simulink model "dynsim_2link_planar"  (R2020a)
settings: Solver=ode3  StartTime=0.0  StopTime=10.0  FixedStep=0.05  RelTol=1e-3
values from neighbouring files (symbols this model uses):
  L1 = 0.337    [dynsim_test_urdf_init.m]    (also in init_2link_planar.m)
  L2 = 0.210    (= 0.21)    [dynsim_test_urdf_init.m]    (also in init_2link_planar.m)
  L3 = 0.268    [dynsim_test_urdf_init.m]    (also in init_2link_planar.m)
  L4 = 0    [dynsim_test_urdf_init.m]    (also in init_2link_planar.m)
  L5 = 0.174    [dynsim_test_urdf_init.m]    (also in init_2link_planar.m)
  L6 = 0    [dynsim_test_urdf_init.m]    (also in init_2link_planar.m)
libraries: robotlib x18, robotmaniplib x1
settings Model: Creator=bascetta  LastModifiedBy=giulio
settings OptimizationCC: EnhancedBackFolding=on  PassReuseOutputArgsAs=Individual arguments  ZeroExternalMemoryAtStartup=off  ZeroInternalMemoryAtStartup=off  MaxStackSize=64  OptimizeBlockOrder=speed  DifferentSizesBufferReuse=on  OptimizationCustomize=off  EfficientTunableParamExpr=on
settings DebuggingCC: ParameterTunabilityLossMsg=error
settings HardwareCC: ProdBitPerPointer=32  ProdBitPerSizeT=32  ProdBitPerPtrDiffT=32  ProdLargestAtomicFloat=None  ProdIntDivRoundTo=Undefined  ProdEndianess=Unspecified  ProdWordSize=32  ProdHWDeviceType=Generic->Unspecified (assume 32-bit Generic)
settings RTWCC: SystemTargetFile=ert.tlc  HardwareBoard=Robot Operating System (ROS)  TemplateMakefile=ert_default_tmf  GenerateReport=on  Toolchain=Catkin  IncludeHyperlinkInReport=on  LaunchReport=on  TargetLang=C++  GenerateTraceInfo=on  GenerateTraceReport=on  GenerateTraceReportSl=on  GenerateTraceReportSf=on  GenerateTraceReportEml=on
settings CodeAppCC: ForceParamTrailComments=on  IgnoreCustomStorageClasses=off  OperatorAnnotations=on  SimulinkDataObjDesc=on  SFDataObjDesc=on  InsertBlockDesc=on
settings ERTTargetCC: SupportContinuousTime=on  SupportVariableSizeSignals=on

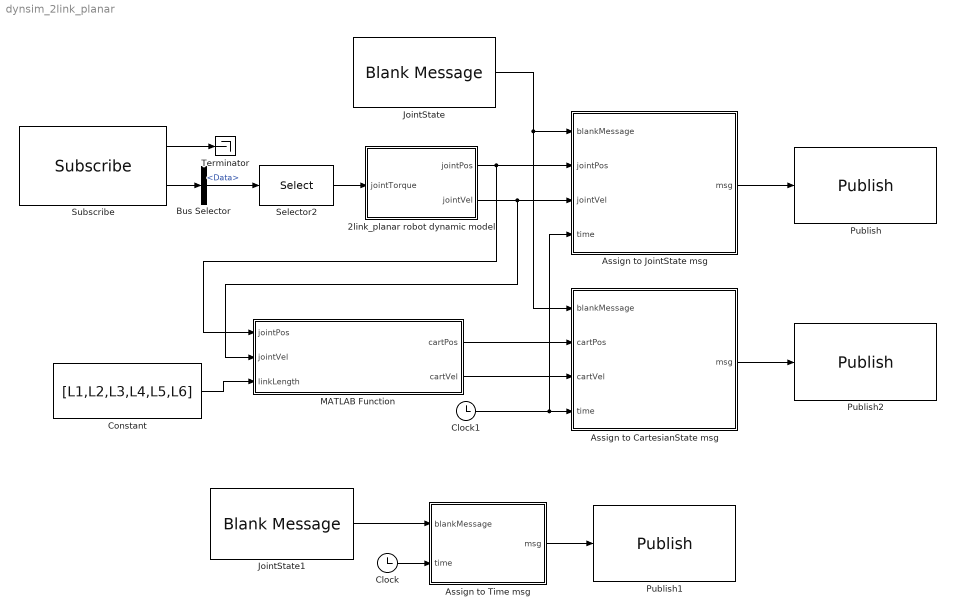
== system dynsim_2link_planar ==
  2link_planar robot dynamic model : Subsystem
  Assign to CartesianState msg : MATLAB Function  TreatAsAtomicUnit=on
  Assign to JointState msg : MATLAB Function  TreatAsAtomicUnit=on
  Assign to Time msg : MATLAB Function  TreatAsAtomicUnit=on
  Bus Selector : BusSelector  OutputSignals=Data
  Clock : Clock
  Clock1 : Clock
  Constant : Constant  Value=[L1,L2,L3,L4,L5,L6]
  JointState : robotlib/Blank Message  messageClass=Message  entityType=sensor_msgs/JointState  messageType=sensor_msgs/JointState  SampleTime=inf
  JointState1 : robotlib/Blank Message  messageClass=Message  entityType=rosgraph_msgs/Clock  messageType=rosgraph_msgs/Clock  SampleTime=inf
  MATLAB Function : MATLAB Function  TreatAsAtomicUnit=on
  Publish : robotlib/Publish  topicSource=Specify your own  topic=/edo/joint_states  messageType=sensor_msgs/JointState  messageQueueLength=1
  Publish1 : robotlib/Publish  topicSource=Specify your own  topic=/clock  messageType=rosgraph_msgs/Clock  messageQueueLength=1
  Publish2 : robotlib/Publish  topicSource=Specify your own  topic=/cartesian_states  messageType=sensor_msgs/JointState  messageQueueLength=1
  Selector2 : Selector  IndexOptions=Starting index (dialog)  Indices=[2]  OutputSizes=6
  Subscribe : robotlib/Subscribe  topicSource=Specify your own  topic=/joint_torque  messageType=std_msgs/Float64MultiArray  sampleTime=-1  messageQueueLength=1
  Terminator : Terminator
  wires:
  JointState1/1 -> Assign to Time msg/1(blankMessage)
  Assign to Time msg/1(msg) -> Publish1/1
  Subscribe/2 -> Bus Selector/1
  Subscribe/1 -> Terminator/1
  Selector2/1 -> 2link_planar robot dynamic model/1(jointTorque)
  Assign to JointState msg/1(msg) -> Publish/1
  2link_planar robot dynamic model/2(jointVel) -> MATLAB Function/2(jointVel), Assign to JointState msg/3(jointVel)
  Bus Selector/1 -> Selector2/1  "<Data>"
  2link_planar robot dynamic model/1(jointPos) -> MATLAB Function/1(jointPos), Assign to JointState msg/2(jointPos)
  Clock/1 -> Assign to Time msg/2(time)
  Clock1/1 -> Assign to CartesianState msg/4(time), Assign to JointState msg/4(time)
  MATLAB Function/2(cartVel) -> Assign to CartesianState msg/3(cartVel)
  Assign to CartesianState msg/1(msg) -> Publish2/1
  Constant/1 -> MATLAB Function/3(linkLength)
  MATLAB Function/1(cartPos) -> Assign to CartesianState msg/2(cartPos)
  JointState/1 -> Assign to CartesianState msg/1(blankMessage), Assign to JointState msg/1(blankMessage)

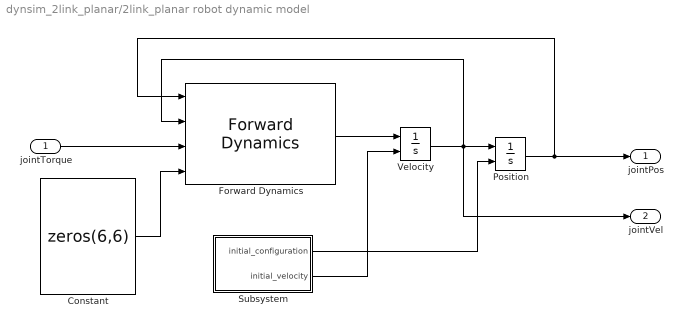
== system dynsim_2link_planar/2link_planar robot dynamic model ==
  jointTorque : Inport
  Constant : Constant  Value=zeros(6,6)
  Forward Dynamics : robotmaniplib/Forward Dynamics  RigidBodyTree=robot_2link_planar  SimulateUsing=Interpreted execution
  Position : Integrator  InitialConditionSource=external
  Subsystem : Subsystem
  Velocity : Integrator  InitialConditionSource=external
  jointPos : Outport
  jointVel : Outport  Port=2
  wires:
  Forward Dynamics/1 -> Velocity/1
  Position/1 -> Forward Dynamics/1, jointPos/1
  jointTorque/1 -> Forward Dynamics/3
  Constant/1 -> Forward Dynamics/4
  Velocity/1 -> Forward Dynamics/2, Position/1, jointVel/1
  Subsystem/2(initial_velocity) -> Velocity/2
  Subsystem/1(initial_configuration) -> Position/2

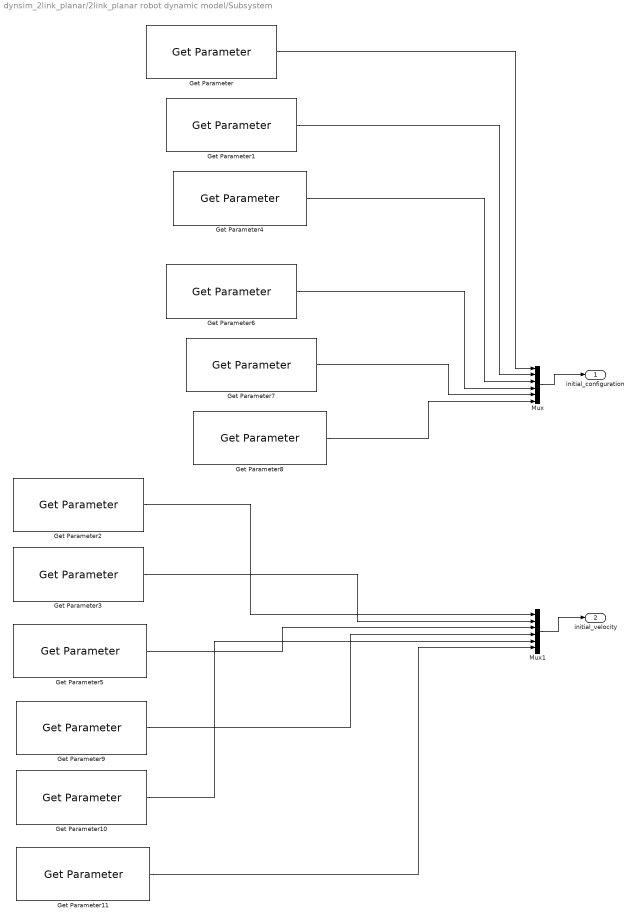
== system dynsim_2link_planar/2link_planar robot dynamic model/Subsystem ==
  Get Parameter : robotlib/Get Parameter  ParameterSource=Specify your own  ParameterName=/dynsim_2link_planar/q1_initial  ParameterType=double  ParameterMaxArrayLength=16  ParameterInitialValue=0  SampleTime=-1  ShowErrorCodeOutput=off  ModelName=dynsim_2link_planar  BlockId=ParamGet_dynsim_2link_planar_112
      settings: SourceProductBaseCode=RR
  Get Parameter1 : robotlib/Get Parameter  ParameterSource=Specify your own  ParameterName=/dynsim_2link_planar/q2_initial  ParameterType=double  ParameterMaxArrayLength=16  ParameterInitialValue=0  SampleTime=-1  ShowErrorCodeOutput=off  ModelName=dynsim_2link_planar  BlockId=ParamGet_dynsim_2link_planar_113
      settings: SourceProductBaseCode=RR
  Get Parameter10 : robotlib/Get Parameter  ParameterSource=Specify your own  ParameterName=/dynnsim_2link_planar/qv5_initial  ParameterType=double  ParameterMaxArrayLength=16  ParameterInitialValue=0  SampleTime=-1  ShowErrorCodeOutput=off  ModelName=dynsim_2link_planar  BlockId=ParamGet_dynsim_2link_planar_135
      settings: SourceProductBaseCode=RR
  Get Parameter11 : robotlib/Get Parameter  ParameterSource=Specify your own  ParameterName=/dynsim_2link_planar/qv5_initial  ParameterType=double  ParameterMaxArrayLength=16  ParameterInitialValue=0  SampleTime=-1  ShowErrorCodeOutput=off  ModelName=dynsim_2link_planar  BlockId=ParamGet_dynsim_2link_planar_136
      settings: SourceProductBaseCode=RR
  Get Parameter2 : robotlib/Get Parameter  ParameterSource=Specify your own  ParameterName=/dynsim_2link_planar/qv1_initial  ParameterType=double  ParameterMaxArrayLength=16  ParameterInitialValue=0  SampleTime=-1  ShowErrorCodeOutput=off  ModelName=dynsim_2link_planar  BlockId=ParamGet_dynsim_2link_planar_117
      settings: SourceProductBaseCode=RR
  Get Parameter3 : robotlib/Get Parameter  ParameterSource=Specify your own  ParameterName=/dynnsim_2link_planar/qv2_initial  ParameterType=double  ParameterMaxArrayLength=16  ParameterInitialValue=0  SampleTime=-1  ShowErrorCodeOutput=off  ModelName=dynsim_2link_planar  BlockId=ParamGet_dynsim_2link_planar_118
      settings: SourceProductBaseCode=RR
  Get Parameter4 : robotlib/Get Parameter  ParameterSource=Specify your own  ParameterName=/dynsim_2link_planar/q3_initial  ParameterType=double  ParameterMaxArrayLength=16  ParameterInitialValue=0  SampleTime=-1  ShowErrorCodeOutput=off  ModelName=dynsim_2link_planar  BlockId=ParamGet_dynsim_2link_planar_129
      settings: SourceProductBaseCode=RR
  Get Parameter5 : robotlib/Get Parameter  ParameterSource=Specify your own  ParameterName=/dynsim_2link_planar/qv3_initial  ParameterType=double  ParameterMaxArrayLength=16  ParameterInitialValue=0  SampleTime=-1  ShowErrorCodeOutput=off  ModelName=dynsim_2link_planar  BlockId=ParamGet_dynsim_2link_planar_130
      settings: SourceProductBaseCode=RR
  Get Parameter6 : robotlib/Get Parameter  ParameterSource=Specify your own  ParameterName=/dynsim_2link_planar/q4_initial  ParameterType=double  ParameterMaxArrayLength=16  ParameterInitialValue=0  SampleTime=-1  ShowErrorCodeOutput=off  ModelName=dynsim_2link_planar  BlockId=ParamGet_dynsim_2link_planar_131
      settings: SourceProductBaseCode=RR
  Get Parameter7 : robotlib/Get Parameter  ParameterSource=Specify your own  ParameterName=/dynsim_2link_planar/q5_initial  ParameterType=double  ParameterMaxArrayLength=16  ParameterInitialValue=0  SampleTime=-1  ShowErrorCodeOutput=off  ModelName=dynsim_2link_planar  BlockId=ParamGet_dynsim_2link_planar_132
      settings: SourceProductBaseCode=RR
  Get Parameter8 : robotlib/Get Parameter  ParameterSource=Specify your own  ParameterName=/dynsim_2link_planar/q6_initial  ParameterType=double  ParameterMaxArrayLength=16  ParameterInitialValue=0  SampleTime=-1  ShowErrorCodeOutput=off  ModelName=dynsim_2link_planar  BlockId=ParamGet_dynsim_2link_planar_133
      settings: SourceProductBaseCode=RR
  Get Parameter9 : robotlib/Get Parameter  ParameterSource=Specify your own  ParameterName=/dynsim_2link_planar/qv4_initial  ParameterType=double  ParameterMaxArrayLength=16  ParameterInitialValue=0  SampleTime=-1  ShowErrorCodeOutput=off  ModelName=dynsim_2link_planar  BlockId=ParamGet_dynsim_2link_planar_134
      settings: SourceProductBaseCode=RR
  Mux : Mux  Inputs=6
  Mux1 : Mux  Inputs=6
  initial_configuration : Outport
  initial_velocity : Outport  Port=2
  wires:
  Mux/1 -> initial_configuration/1
  Get Parameter/1 -> Mux/1
  Get Parameter1/1 -> Mux/2
  Get Parameter3/1 -> Mux1/2
  Get Parameter2/1 -> Mux1/1
  Mux1/1 -> initial_velocity/1
  Get Parameter4/1 -> Mux/3
  Get Parameter5/1 -> Mux1/3
  Get Parameter6/1 -> Mux/4
  Get Parameter7/1 -> Mux/5
  Get Parameter8/1 -> Mux/6
  Get Parameter9/1 -> Mux1/4
  Get Parameter10/1 -> Mux1/5
  Get Parameter11/1 -> Mux1/6

== matlab function dynsim_2link_planar/Assign to Time msg ==
  data: blankMessage input Bus: SL_Bus_dynsim_2link_planar_rosgraph_msgs_Clock; msg output Bus: SL_Bus_dynsim_2link_planar_rosgraph_msgs_Clock; time input
function msg = assign_Time(blankMessage,time)
%#codegen

% Assign the output message to be the same with input blank message
msg = blankMessage;

% Convert and set time
msg.Clock_.Sec  = fix(time);
msg.Clock_.Nsec = fix((time-fix(time))*1e9);

== matlab function dynsim_2link_planar/Assign to JointState msg ==
  data: blankMessage input; msg output Bus: SL_Bus_dynsim_2link_planar_sensor_msgs_JointState; jointPos input; jointVel input; time input
function msg = assign_JointState(blankMessage,jointPos,jointVel,time)
%#codegen

% Assign the output message to be the same with input blank message
msg = blankMessage;

% Initialize time stamp
msg.Header.Stamp.Sec  = fix(time);
msg.Header.Stamp.Nsec = fix((time-fix(time))*1e9);

% Set the number of strings in the string array, and joint positions/velocities in the position/velocity array
numJoints = length(jointPos);
msg.Name_SL_Info.CurrentLength = uint32(numJoints);
msg.Position_SL_Info.CurrentLength = uint32(numJoints);
msg.Velocity_SL_Info.CurrentLength = uint32(numJoints);

% Set the individual components in the message arrays
strArrayToAssign = {'edo_joint_1', 'edo_joint_2', 'edo_joint_3', 'edo_joint_4', 'edo_joint_5', 'edo_joint_6'};

for idx=1:numJoints
    str = strArrayToAssign{idx};
    strLength = length(str);
    msg.Name(idx).Data(1:strLength) = uint8(str);
    msg.Name(idx).Data_SL_Info.CurrentLength = uint32(strLength);

    msg.Position(idx) = jointPos(idx);
    msg.Velocity(idx) = jointVel(idx);
end

== matlab function dynsim_2link_planar/MATLAB Function ==
  data: jointPos input; cartPos output; jointVel input; cartVel output; linkLength input
function [cartPos, cartVel] = forward_kinematics_2link(jointPos,jointVel,linkLength)

cartPos = zeros(1,3);
cartVel = zeros(1,3);

L1 = linkLength(1);
L2 = linkLength(2);
L3 = linkLength(3);
L4 = linkLength(4);
L5 = linkLength(5);
L6 = linkLength(6);
q1 = jointPos(1);
q2 = jointPos(2);
q3 = jointPos(3);
q4 = jointPos(4);
q5 = jointPos(5);
q6 = jointPos(6);
qv1 = jointVel(1);
qv2 = jointVel(2);
qv3 = jointVel(3);
qv4 = jointVel(4);
qv5 = jointVel(5);
qv6 = jointVel(6);

cartPos(1) = (21*cos(q1)*cos(q2))/100 - (881990442724166438595063481850742017710301237698608276441511348391*sin(q3)*(cos(q1)*cos(q2) - (4967757600021511*sin(q1)*sin(q2))/81129638414606681695789005144064))/3291009114642412084309938365114701009965471731267159726697218048000 - (4381514724989315025408999478707104134677774883409634064639353719090171372215238801*sin(q1))/266998379490113760299377713271194014325338065294581596243380200977777465722580068752870260867072000 - (104322909600451731*sin(q1)*sin(q2))/8112963841460668169578900514406400 - (432194911201871457*cos(q4)*((4967757600021511*sin(q3)*(cos(q1)*cos(q2) - (4967757600021511*sin(q1)*sin(q2))/81129638414606681695789005144064))/81129638414606681695789005144064 - sin(q1) + (4967757600021511*cos(q3)*(cos(q1)*sin(q2) + (4967757600021511*cos(q2)*sin(q1))/81129638414606681695789005144064))/81129638414606681695789005144064))/40564819207303340847894502572032000 + (87*cos(q5)*((4967757600021511*sin(q1))/81129638414606681695789005144064 + sin(q3)*(cos(q1)*cos(q2) - (4967757600021511*sin(q1)*sin(q2))/81129638414606681695789005144064) - (4967757600021511*cos(q4)*((4967757600021511*sin(q3)*(cos(q1)*cos(q2) - (4967757600021511*sin(q1)*sin(q2))/81129638414606681695789005144064))/81129638414606681695789005144064 - sin(q1) + (4967757600021511*cos(q3)*(cos(q1)*sin(q2) + (4967757600021511*cos(q2)*sin(q1))/81129638414606681695789005144064))/81129638414606681695789005144064))/81129638414606681695789005144064 + (4967757600021511*sin(q4)*(sin(q3)*(cos(q1)*sin(q2) + (4967757600021511*cos(q2)*sin(q1))/81129638414606681695789005144064) - cos(q3)*(cos(q1)*cos(q2) - (4967757600021511*sin(q1)*sin(q2))/81129638414606681695789005144064)))/81129638414606681695789005144064 + cos(q3)*(cos(q1)*sin(q2) + (4967757600021511*cos(q2)*sin(q1))/81129638414606681695789005144064)))/500 + (87*sin(q5)*(sin(q4)*((4967757600021511*sin(q3)*(cos(q1)*cos(q2) - (4967757600021511*sin(q1)*sin(q2))/81129638414606681695789005144064))/81129638414606681695789005144064 - sin(q1) + (4967757600021511*cos(q3)*(cos(q1)*sin(q2) + (4967757600021511*cos(q2)*sin(q1))/81129638414606681695789005144064))/81129638414606681695789005144064) + cos(q4)*(sin(q3)*(cos(q1)*sin(q2) + (4967757600021511*cos(q2)*sin(q1))/81129638414606681695789005144064) - cos(q3)*(cos(q1)*cos(q2) - (4967757600021511*sin(q1)*sin(q2))/81129638414606681695789005144064))))/500 + (432194911201871457*sin(q4)*(sin(q3)*(cos(q1)*sin(q2) + (4967757600021511*cos(q2)*sin(q1))/81129638414606681695789005144064) - cos(q3)*(cos(q1)*cos(q2) - (4967757600021511*sin(q1)*sin(q2))/81129638414606681695789005144064)))/40564819207303340847894502572032000 - (881990442724166438595063481850742017710301237698608276441511348391*cos(q3)*(cos(q1)*sin(q2) + (4967757600021511*cos(q2)*sin(q1))/81129638414606681695789005144064))/3291009114642412084309938365114701009965471731267159726697218048000
cartPos(2) = (4381514724989315025408999478707104134677774883409634064639353719090171372215238801*cos(q1))/266998379490113760299377713271194014325338065294581596243380200977777465722580068752870260867072000 - (881990442724166438595063481850742017710301237698608276441511348391*sin(q3)*((4967757600021511*cos(q1)*sin(q2))/81129638414606681695789005144064 + cos(q2)*sin(q1)))/3291009114642412084309938365114701009965471731267159726697218048000 - (87*sin(q5)*(cos(q4)*(sin(q3)*((4967757600021511*cos(q1)*cos(q2))/81129638414606681695789005144064 - sin(q1)*sin(q2)) + cos(q3)*((4967757600021511*cos(q1)*sin(q2))/81129638414606681695789005144064 + cos(q2)*sin(q1))) - sin(q4)*(cos(q1) + (4967757600021511*sin(q3)*((4967757600021511*cos(q1)*sin(q2))/81129638414606681695789005144064 + cos(q2)*sin(q1)))/81129638414606681695789005144064 - (4967757600021511*cos(q3)*((4967757600021511*cos(q1)*cos(q2))/81129638414606681695789005144064 - sin(q1)*sin(q2)))/81129638414606681695789005144064)))/500 + (104322909600451731*cos(q1)*sin(q2))/8112963841460668169578900514406400 + (21*cos(q2)*sin(q1))/100 - (432194911201871457*sin(q4)*(sin(q3)*((4967757600021511*cos(q1)*cos(q2))/81129638414606681695789005144064 - sin(q1)*sin(q2)) + cos(q3)*((4967757600021511*cos(q1)*sin(q2))/81129638414606681695789005144064 + cos(q2)*sin(q1))))/40564819207303340847894502572032000 - (87*cos(q5)*((4967757600021511*cos(q1))/81129638414606681695789005144064 - sin(q3)*((4967757600021511*cos(q1)*sin(q2))/81129638414606681695789005144064 + cos(q2)*sin(q1)) + (4967757600021511*sin(q4)*(sin(q3)*((4967757600021511*cos(q1)*cos(q2))/81129638414606681695789005144064 - sin(q1)*sin(q2)) + cos(q3)*((4967757600021511*cos(q1)*sin(q2))/81129638414606681695789005144064 + cos(q2)*sin(q1))))/81129638414606681695789005144064 + (4967757600021511*cos(q4)*(cos(q1) + (4967757600021511*sin(q3)*((4967757600021511*cos(q1)*sin(q2))/81129638414606681695789005144064 + cos(q2)*sin(q1)))/81129638414606681695789005144064 - (4967757600021511*cos(q3)*((4967757600021511*cos(q1)*cos(q2))/81129638414606681695789005144064 - sin(q1)*sin(q2)))/81129638414606681695789005144064))/81129638414606681695789005144064 + cos(q3)*((4967757600021511*cos(q1)*cos(q2))/81129638414606681695789005144064 - sin(q1)*sin(q2))))/500 - (432194911201871457*cos(q4)*(cos(q1) + (4967757600021511*sin(q3)*((4967757600021511*cos(q1)*sin(q2))/81129638414606681695789005144064 + cos(q2)*sin(q1)))/81129638414606681695789005144064 - (4967757600021511*cos(q3)*((4967757600021511*cos(q1)*cos(q2))/81129638414606681695789005144064 - sin(q1)*sin(q2)))/81129638414606681695789005144064))/40564819207303340847894502572032000 + (881990442724166438595063481850742017710301237698608276441511348391*cos(q3)*((4967757600021511*cos(q1)*cos(q2))/81129638414606681695789005144064 - sin(q1)*sin(q2)))/3291009114642412084309938365114701009965471731267159726697218048000
cartPos(3) = (67*sin(q2)*sin(q3))/250 - (67*cos(q2)*cos(q3))/250 - (21*sin(q2))/100 - (87*cos(q5)*(sin(q2)*sin(q3) - cos(q2)*cos(q3) + (4967757600021511*cos(q4)*((4967757600021511*cos(q2)*cos(q3))/81129638414606681695789005144064 - (4967757600021511*sin(q2)*sin(q3))/81129638414606681695789005144064 + 4967757600021511/81129638414606681695789005144064))/81129638414606681695789005144064 - (4967757600021511*sin(q4)*(cos(q2)*sin(q3) + cos(q3)*sin(q2)))/81129638414606681695789005144064 + 684969180613545/182687704666362864775460604089535377456991567872))/500 - (3376522743764621*cos(q4)*((4967757600021511*cos(q2)*cos(q3))/81129638414606681695789005144064 - (4967757600021511*sin(q2)*sin(q3))/81129638414606681695789005144064 + 4967757600021511/81129638414606681695789005144064))/316912650057057350374175801344000 + (3376522743764621*sin(q4)*(cos(q2)*sin(q3) + cos(q3)*sin(q2)))/316912650057057350374175801344000 + (87*sin(q5)*(sin(q4)*((4967757600021511*cos(q2)*cos(q3))/81129638414606681695789005144064 - (4967757600021511*sin(q2)*sin(q3))/81129638414606681695789005144064 + 4967757600021511/81129638414606681695789005144064) + cos(q4)*(cos(q2)*sin(q3) + cos(q3)*sin(q2))))/500 + 337/1000

cartVel(1) = (87*cos(q5)*(sin(q4)*(sin(q3)*((4967757600021511*cos(q1)*cos(q2))/81129638414606681695789005144064 - sin(q1)*sin(q2)) + cos(q3)*((4967757600021511*cos(q1)*sin(q2))/81129638414606681695789005144064 + cos(q2)*sin(q1))) + cos(q4)*((4967757600021511*sin(q3)*((4967757600021511*cos(q1)*sin(q2))/81129638414606681695789005144064 + cos(q2)*sin(q1)))/81129638414606681695789005144064 - (4967757600021511*cos(q3)*((4967757600021511*cos(q1)*cos(q2))/81129638414606681695789005144064 - sin(q1)*sin(q2)))/81129638414606681695789005144064)))/500 - (87*sin(q5)*((4967757600021511*sin(q4)*((4967757600021511*sin(q3)*((4967757600021511*cos(q1)*sin(q2))/81129638414606681695789005144064 + cos(q2)*sin(q1)))/81129638414606681695789005144064 - (4967757600021511*cos(q3)*((4967757600021511*cos(q1)*cos(q2))/81129638414606681695789005144064 - sin(q1)*sin(q2)))/81129638414606681695789005144064))/81129638414606681695789005144064 - (4967757600021511*cos(q4)*(sin(q3)*((4967757600021511*cos(q1)*cos(q2))/81129638414606681695789005144064 - sin(q1)*sin(q2)) + cos(q3)*((4967757600021511*cos(q1)*sin(q2))/81129638414606681695789005144064 + cos(q2)*sin(q1))))/81129638414606681695789005144064))/500
cartVel(2) = (87*cos(q5)*(sin(q4)*(sin(q3)*(cos(q1)*sin(q2) + (4967757600021511*cos(q2)*sin(q1))/81129638414606681695789005144064) - cos(q3)*(cos(q1)*cos(q2) - (4967757600021511*sin(q1)*sin(q2))/81129638414606681695789005144064)) - cos(q4)*((4967757600021511*sin(q3)*(cos(q1)*cos(q2) - (4967757600021511*sin(q1)*sin(q2))/81129638414606681695789005144064))/81129638414606681695789005144064 + (4967757600021511*cos(q3)*(cos(q1)*sin(q2) + (4967757600021511*cos(q2)*sin(q1))/81129638414606681695789005144064))/81129638414606681695789005144064)))/500 + (87*sin(q5)*((4967757600021511*sin(q4)*((4967757600021511*sin(q3)*(cos(q1)*cos(q2) - (4967757600021511*sin(q1)*sin(q2))/81129638414606681695789005144064))/81129638414606681695789005144064 + (4967757600021511*cos(q3)*(cos(q1)*sin(q2) + (4967757600021511*cos(q2)*sin(q1))/81129638414606681695789005144064))/81129638414606681695789005144064))/81129638414606681695789005144064 + (4967757600021511*cos(q4)*(sin(q3)*(cos(q1)*sin(q2) + (4967757600021511*cos(q2)*sin(q1))/81129638414606681695789005144064) - cos(q3)*(cos(q1)*cos(q2) - (4967757600021511*sin(q1)*sin(q2))/81129638414606681695789005144064)))/81129638414606681695789005144064))/500
cartVel(3) = (87*sin(q5)*((4967757600021511*sin(q4)*((4967757600021511*cos(q2)*cos(q3))/81129638414606681695789005144064 - (4967757600021511*sin(q2)*sin(q3))/81129638414606681695789005144064))/81129638414606681695789005144064 + (4967757600021511*cos(q4)*(cos(q2)*sin(q3) + cos(q3)*sin(q2)))/81129638414606681695789005144064))/500 - (87*cos(q5)*(cos(q4)*((4967757600021511*cos(q2)*cos(q3))/81129638414606681695789005144064 - (4967757600021511*sin(q2)*sin(q3))/81129638414606681695789005144064) - sin(q4)*(cos(q2)*sin(q3) + cos(q3)*sin(q2))))/500

== matlab function dynsim_2link_planar/Assign to CartesianState msg ==
  data: blankMessage input; msg output Bus: SL_Bus_dynsim_2link_planar_sensor_msgs_JointState; cartPos input; cartVel input; time input
function msg = assign_CartesianState(blankMessage,cartPos,cartVel,time)
%#codegen

% Assign the output message to be the same with input blank message
msg = blankMessage;

% Initialize time stamp
msg.Header.Stamp.Sec  = fix(time);
msg.Header.Stamp.Nsec = fix((time-fix(time))*1e9);

% Set the number of strings in the string array, and joint positions/velocities in the position/velocity array
numCoordinates = length(cartPos);
msg.Name_SL_Info.CurrentLength = uint32(numCoordinates);
msg.Position_SL_Info.CurrentLength = uint32(numCoordinates);
msg.Velocity_SL_Info.CurrentLength = uint32(numCoordinates);

% Set the individual components in the message arrays
strArrayToAssign = {'edo_joint_1', 'edo_joint_2', 'edo_joint_3', 'edo_joint_4', 'edo_joint_5', 'edo_joint_6'};

for idx=1:numCoordinates
    str = strArrayToAssign{idx};
    strLength = length(str);
    msg.Name(idx).Data(1:strLength) = uint8(str);
    msg.Name(idx).Data_SL_Info.CurrentLength = uint32(strLength);

    msg.Position(idx) = cartPos(idx);
    msg.Velocity(idx) = cartVel(idx);
end
